simulink model "leaderless_consensus_control"  (R2023a)
settings: Solver=VariableStepAuto  StartTime=0.0  StopTime=10.0  RelTol=1e-3
values from neighbouring files (symbols this model uses):
  A_bar = kron(eye(N),A)    [leaderless_consensus.m]
  B_bar = kron(eye(N),B)    [leaderless_consensus.m]
  Cf_bar = kron(eye(N), Cf)    [leaderless_consensus.m]
  Df_bar = kron(eye(N),Df)    [leaderless_consensus.m]
  k = lqr(A,B,Q,R)    [leaderless_consensus.m]
  L = [2 -1 -1;-1 2 -1;-1 -1 2]    [leaderless_consensus.m]
  n = 2    [leaderless_consensus.m]
  N = 3    [leaderless_consensus.m]
settings Model: Creator=BALA SUBRAHMANYAM  LastModifiedBy=BALA SUBRAHMANYAM

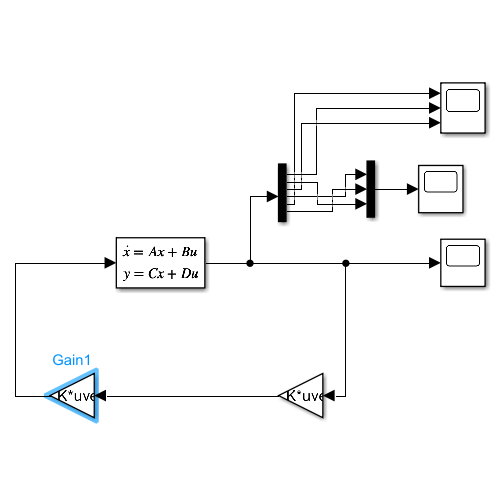
[thumbnail: Simulink's stored preview of the top-level diagram]
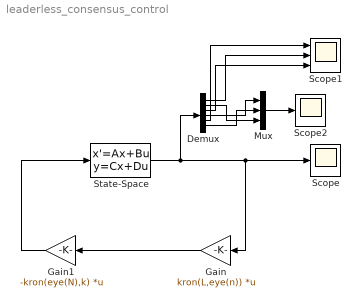
== system leaderless_consensus_control ==
  Demux : Demux  Outputs=6
  Gain : Gain  Gain=kron(L,eye(n))  Multiplication=Matrix(K*u) (u vector)
  Gain1 : Gain  Gain=-kron(eye(N),k)  Multiplication=Matrix(K*u) (u vector)
  Mux : Mux  Inputs=3
  Scope : Scope
  Scope1 : Scope  NumInputPorts=3
  Scope2 : Scope
  State-Space : StateSpace  A=A_bar  B=B_bar  C=Cf_bar  D=Df_bar  InitialCondition=[-1;2;1;4;2;6]  ParameterTunability=Unconstrained
  wires:
  Gain/1 -> Gain1/1
  Gain1/1 -> State-Space/1
  State-Space/1 -> Demux/1, Scope/1, Gain/1
  Demux/1 -> Scope1/2
  Demux/3 -> Scope1/3
  Demux/6 -> Mux/2
  Demux/4 -> Mux/1
  Demux/2 -> Mux/3
  Demux/5 -> Scope1/1
  Mux/1 -> Scope2/1
